simulink model "EKF_IMU_DVL_MAP"  (R2015a)
settings: Solver=ode45  StartTime=0.0  StopTime=t_simulation  RelTol=1e-3
InitFcn:
  | launch_sim
settings Model: Creator=Adrien  LastModifiedBy=Adrien

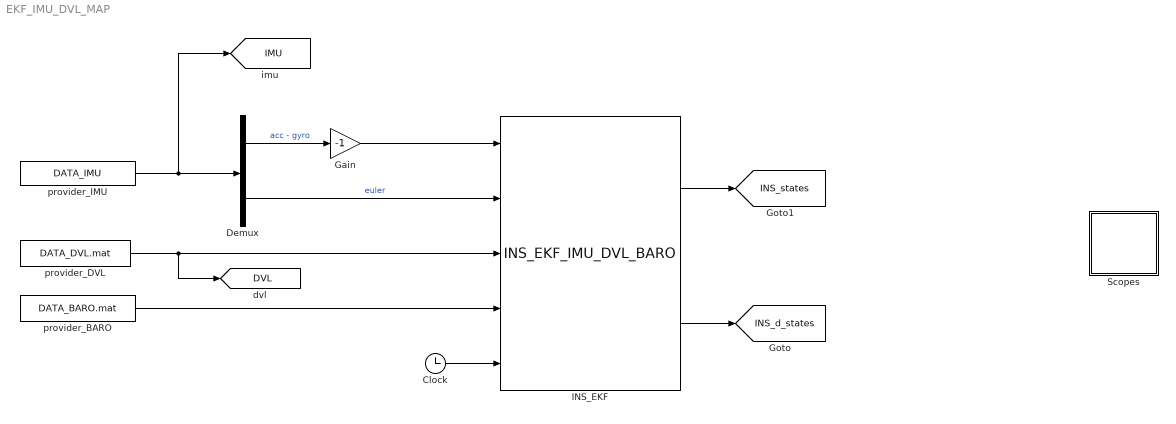
== system EKF_IMU_DVL_MAP ==
  Clock : Clock
  Demux : Demux  Outputs=[6, 3]
  Gain : Gain  Gain=-1
  INS_EKF : M-S-Function  FunctionName=INS_EKF_IMU_DVL_BARO
  Scopes : Subsystem
  provider_BARO : FromFile  FileName=DATA_BARO.mat
  provider_DVL : FromFile  FileName=DATA_DVL.mat
  provider_IMU : FromFile  FileName=DATA_IMU
  tag scope: DVL=global, IMU=global, INS_d_states=global, INS_states=global
  wires:
  Demux/1 -> Gain/1  "acc - gyro"
  Demux/2 -> INS_EKF/2  "euler"
  provider_BARO/1 -> INS_EKF/4
  Clock/1 -> INS_EKF/5
  INS_EKF/2 -> [INS_d_states]
  INS_EKF/1 -> [INS_states]
  provider_IMU/1 -> [IMU], Demux/1
  Gain/1 -> INS_EKF/1
  provider_DVL/1 -> INS_EKF/3, [DVL]

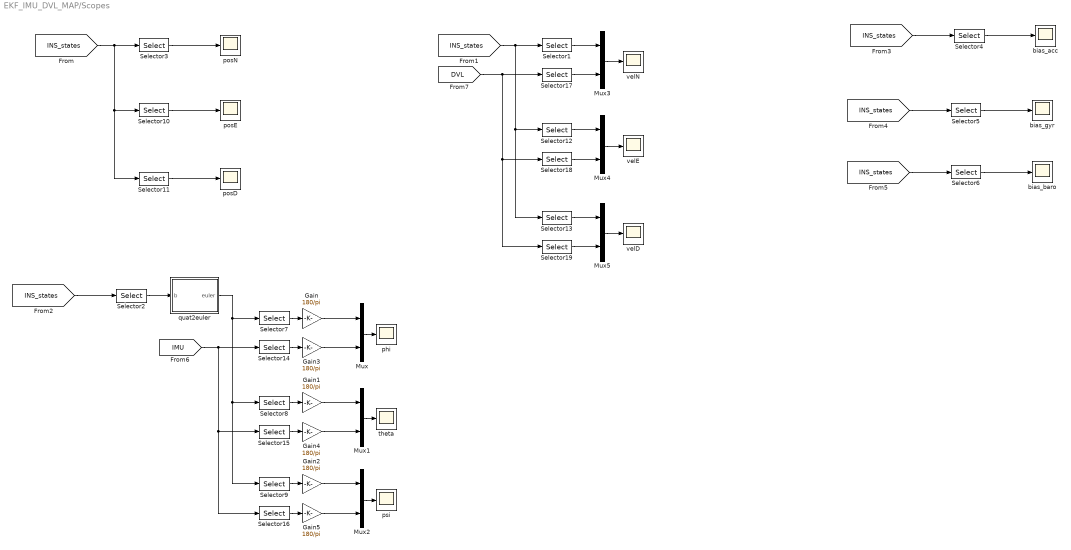
== system EKF_IMU_DVL_MAP/Scopes ==
  Gain{,1..5} (6 alike) : Gain  Gain=180/pi
  Mux{,1..5} (6 alike) : Mux  Inputs=2
  Selector1 : Selector  InputPortWidth=17  Indices=4
  Selector10 : Selector  InputPortWidth=17  Indices=2
  Selector11 : Selector  InputPortWidth=17  Indices=3
  Selector12 : Selector  InputPortWidth=17  Indices=5
  Selector13 : Selector  InputPortWidth=17  Indices=6
  Selector14 : Selector  InputPortWidth=9  Indices=7
  Selector15 : Selector  InputPortWidth=9  Indices=8
  Selector16 : Selector  InputPortWidth=9  Indices=9
  Selector17 : Selector  InputPortWidth=5
  Selector18 : Selector  InputPortWidth=5  Indices=2
  Selector19 : Selector  InputPortWidth=5  Indices=3
  Selector2 : Selector  InputPortWidth=17  Indices=[7:10]
  Selector3 : Selector  InputPortWidth=17
  Selector4 : Selector  InputPortWidth=17  Indices=[11:13]
  Selector5 : Selector  InputPortWidth=17  Indices=[14:16]
  Selector6 : Selector  InputPortWidth=17  Indices=17
  Selector7 : Selector  InputPortWidth=3
  Selector8 : Selector  InputPortWidth=3  Indices=2
  Selector9 : Selector  InputPortWidth=3  Indices=3
  bias_acc : Scope
      settings: SaveName=ScopeData4
  bias_baro : Scope
      settings: SaveName=ScopeData6
  bias_gyr : Scope
      settings: SaveName=ScopeData5
  phi : Scope
      settings: SaveName=ScopeData2
  posD : Scope
      settings: SaveName=ScopeData10
  posE : Scope
      settings: SaveName=ScopeData9
  posN : Scope
      settings: YMin=-0.75  YMax=4.75
  psi : Scope
      settings: SaveName=ScopeData8
  quat2euler : MATLAB Function  TreatAsAtomicUnit=on
  theta : Scope
      settings: YMin=-2  YMax=22  SaveName=ScopeData7
  velD : Scope
      settings: SaveName=ScopeData12
  velE : Scope
      settings: SaveName=ScopeData11
  velN : Scope
  wires:
  [INS_states] -> Selector13/1, Selector12/1, Selector1/1
  Selector2/1 -> quat2euler/1(b)
  [INS_states] -> Selector11/1, Selector10/1, Selector3/1
  Selector3/1 -> posN/1
  [INS_states] -> Selector2/1
  Selector4/1 -> bias_acc/1
  [INS_states] -> Selector4/1
  Selector5/1 -> bias_gyr/1
  [INS_states] -> Selector5/1
  Selector6/1 -> bias_baro/1
  [INS_states] -> Selector6/1
  quat2euler/1(euler) -> Selector9/1, Selector8/1, Selector7/1
  Selector8/1 -> Gain1/1
  Selector9/1 -> Gain2/1
  Selector7/1 -> Gain/1
  Selector10/1 -> posE/1
  Selector11/1 -> posD/1
  Selector14/1 -> Gain3/1
  Gain3/1 -> Mux/2
  Mux/1 -> phi/1
  Gain/1 -> Mux/1
  Mux1/1 -> theta/1
  Mux2/1 -> psi/1
  Gain2/1 -> Mux2/1
  Selector15/1 -> Gain4/1
  Selector16/1 -> Gain5/1
  [IMU] -> Selector15/1, Selector16/1, Selector14/1
  Gain5/1 -> Mux2/2
  Mux3/1 -> velN/1
  Selector1/1 -> Mux3/1
  [DVL] -> Selector19/1, Selector18/1, Selector17/1
  Mux4/1 -> velE/1
  Mux5/1 -> velD/1
  Selector12/1 -> Mux4/1
  Selector13/1 -> Mux5/1
  Selector17/1 -> Mux3/2
  Selector19/1 -> Mux5/2
  Selector18/1 -> Mux4/2
  Gain1/1 -> Mux1/1
  Gain4/1 -> Mux1/2

== matlab function EKF_IMU_DVL_MAP/Scopes/quat2euler ==
  data: b input; euler output
function euler = quat2euler(b)

euler = zeros(3,1);

phi = atan2(2*(b(3)*b(4) - b(1)*b(2)),1 - 2*(b(2)^2 + b(3)^2));
theta = asin(-2*(b(2)*b(4) + b(1)*b(3)));
psi = atan2(2*(b(2)*b(3) - b(1)*b(4)),1 - 2*(b(3)^2 + b(4)^2));

euler(1) = phi;
euler(2) = theta;
euler(3) = psi;
